simulink model "Simulation"  (R2020b)
settings: Solver=VariableStepAuto  StartTime=0.0  StopTime=15  RelTol=1e-3
values from neighbouring files (symbols this model uses):
  Ac = [0 1 0 0 ... (first row only)    [Model_Init.m]
  B1c = [0; 2*cf/m; 0; 2*lf*cf/iz]    [Model_Init.m]
  K = acker(Ac,B1c,kp)    [Model_Init.m]
  n_p = 30    [Model_Init.m]
  Ts = 0.1    [Model_Init.m]
  v0_ego = 13.9    [Model_Init.m]
undefined symbols (not defined in the file or in its folder): DiscIntNeverNeededParam
libraries: simulink x2
settings Model: Creator=Stage  LastModifiedBy=Stage

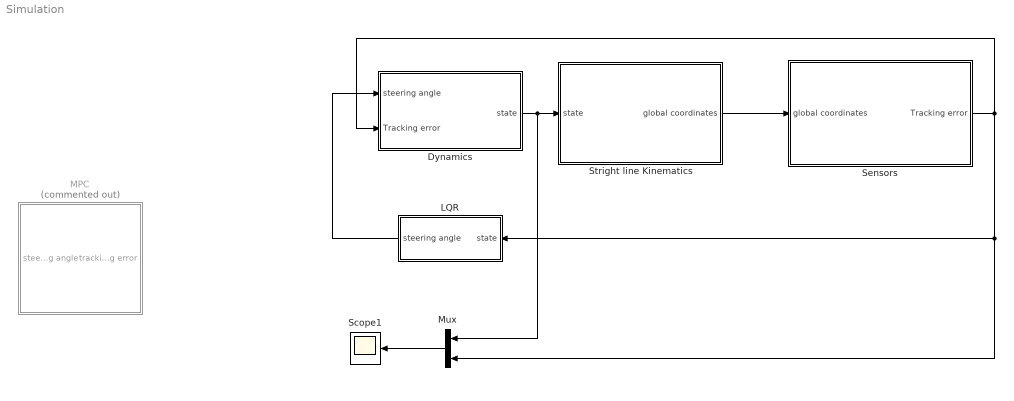
== system Simulation ==
  Dynamics : Subsystem
  "LQR " : Subsystem
  MPC : Subsystem  Commented=on
  Mux : Mux  Inputs=2
  Scope1 : Scope
  Sensors : Subsystem
  Stright line Kinematics : Subsystem
  wires:
  Stright line Kinematics/1(global coordinates) -> Sensors/1(global coordinates)
  Dynamics/1(state) -> Mux/1, Stright line Kinematics/1(state)
  Sensors/1(Tracking error) -> "LQR "/1(state), Mux/2, Dynamics/2(Tracking error)
  "LQR "/1(steering angle) -> Dynamics/1(steering angle)
  Mux/1 -> Scope1/1

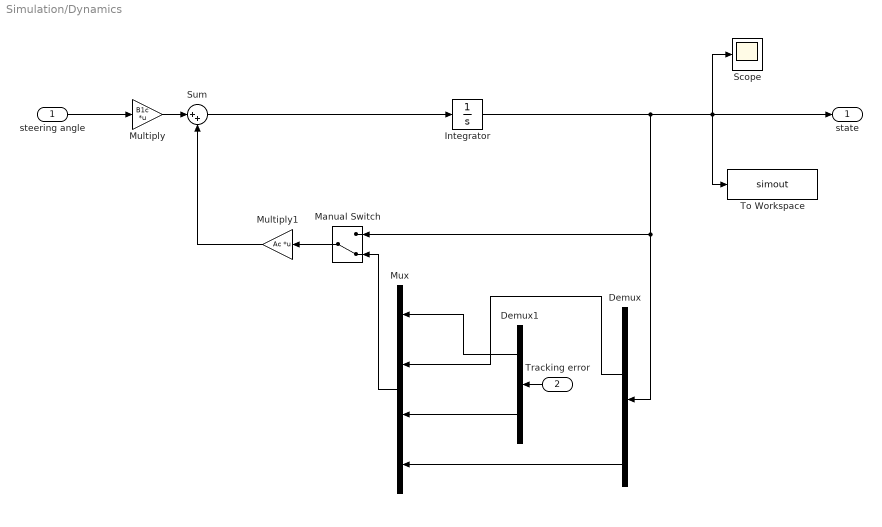
== system Simulation/Dynamics ==
  steering angle : Inport
  Tracking error : Inport  Port=2
  Demux : Demux
  Demux1 : Demux  Outputs=2
  Integrator : Integrator  InitialCondition=[1 0 0 0]
  Manual Switch : ManualSwitch  CurrentSetting=0
  Multiply : Gain  Gain=B1c  Multiplication=Matrix(K*u) (u vector)
  Multiply1 : Gain  Gain=Ac  Multiplication=Matrix(K*u) (u vector)
  Mux : Mux
  Scope : Scope
  Sum : Sum  Inputs=|++
  To Workspace : ToWorkspace  VariableName=simout  SampleTime=-1
  state : Outport
  wires:
  steering angle/1 -> Multiply/1
  Multiply/1 -> Sum/1
  Sum/1 -> Integrator/1
  Multiply1/1 -> Sum/2
  Manual Switch/1 -> Multiply1/1
  Mux/1 -> Manual Switch/2
  Tracking error/1 -> Demux1/1
  Integrator/1 -> Demux/1, Manual Switch/1, Scope/1, state/1, To Workspace/1
  Demux1/1 -> Mux/1
  Demux1/2 -> Mux/3
  Demux/2 -> Mux/2
  Demux/4 -> Mux/4

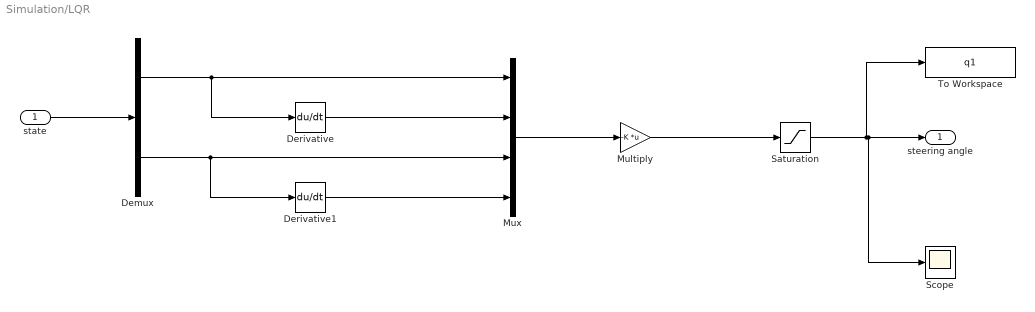
== system Simulation/LQR  ==
  state : Inport
  Demux : Demux  Outputs=2
  Derivative : Derivative
  Derivative1 : Derivative
  Multiply : Gain  Gain=-K  Multiplication=Matrix(K*u) (u vector)
  Mux : Mux
  Saturation : Saturate  UpperLimit=0.3  LowerLimit=-0.3
  Scope : Scope
  To Workspace : ToWorkspace  VariableName=q1  SaveFormat=Timeseries  SampleTime=-1
  steering angle : Outport
  wires:
  Multiply/1 -> Saturation/1
  Saturation/1 -> To Workspace/1, Scope/1, steering angle/1
  state/1 -> Demux/1
  Demux/1 -> Derivative/1, Mux/1
  Demux/2 -> Derivative1/1, Mux/3
  Derivative1/1 -> Mux/4
  Derivative/1 -> Mux/2
  Mux/1 -> Multiply/1

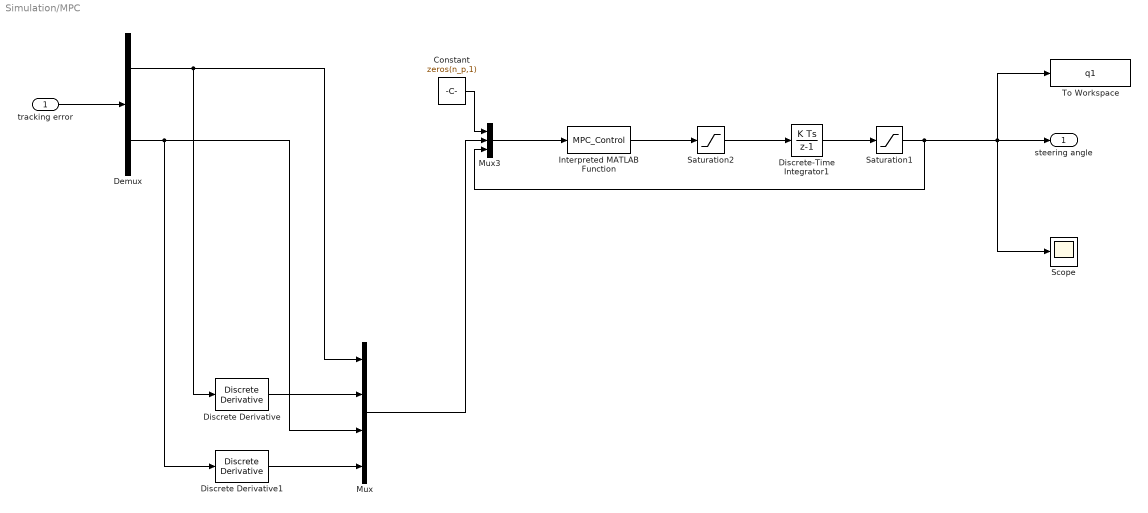
== system Simulation/MPC ==
  tracking error : Inport
  Constant : Constant  Value=zeros(n_p,1)
  Demux : Demux  Outputs=2
  Discrete Derivative : simulink/Discrete/Discrete Derivative  gainval=1.0  ICPrevScaledInput=10  OutMin=[]  OutMax=[]  OutDataType=fixdt(1, 16)  OutScaling=2^-10  DoSatur=off
  Discrete Derivative1 : simulink/Discrete/Discrete Derivative  gainval=1.0  ICPrevScaledInput=0.0  OutMin=[]  OutMax=[]  OutDataType=fixdt(1, 16)  OutScaling=2^-10  DoSatur=off
  Discrete-Time Integrator1 : DiscreteIntegrator  SampleTime=Ts  ICPrevOutput=DiscIntNeverNeededParam  ICPrevScaledInput=DiscIntNeverNeededParam
  Interpreted MATLAB Function : MATLABFcn  MATLABFcn=MPC_Control  OutputDimensions=1
  Mux : Mux
  Mux3 : Mux  Inputs=3
  Saturation1 : Saturate  UpperLimit=0.2  LowerLimit=-0.2
  Saturation2 : Saturate  UpperLimit=0.04  LowerLimit=-0.04
  Scope : Scope
  To Workspace : ToWorkspace  VariableName=q1  SampleTime=-1
  steering angle : Outport
  wires:
  Discrete-Time Integrator1/1 -> Saturation1/1
  Saturation1/1 -> Mux3/3, steering angle/1, Scope/1, To Workspace/1
  Mux3/1 -> Interpreted MATLAB Function/1
  Interpreted MATLAB Function/1 -> Saturation2/1
  Constant/1 -> Mux3/1
  tracking error/1 -> Demux/1
  Demux/1 -> Discrete Derivative/1, Mux/1
  Demux/2 -> Discrete Derivative1/1, Mux/3
  Mux/1 -> Mux3/2
  Discrete Derivative1/1 -> Mux/4
  Discrete Derivative/1 -> Mux/2
  Saturation2/1 -> Discrete-Time Integrator1/1

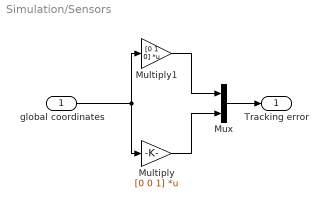
== system Simulation/Sensors ==
  global coordinates : Inport
  Multiply : Gain  Gain=[0 0 1]  Multiplication=Matrix(K*u) (u vector)
  Multiply1 : Gain  Gain=[0 1 0]  Multiplication=Matrix(K*u) (u vector)
  Mux : Mux  Inputs=2
  Tracking error : Outport
  wires:
  global coordinates/1 -> Multiply1/1, Multiply/1
  Multiply/1 -> Mux/2
  Multiply1/1 -> Mux/1
  Mux/1 -> Tracking error/1

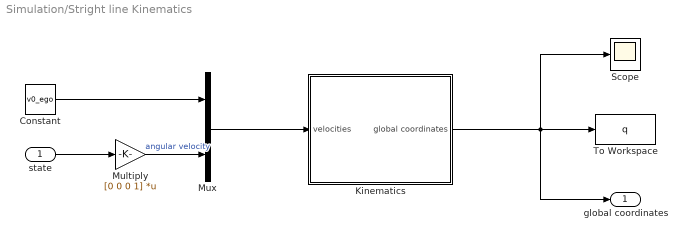
== system Simulation/Stright line Kinematics ==
  state : Inport
  Constant : Constant  Value=v0_ego
  "Kinematics " : Subsystem
  Multiply : Gain  Gain=[0 0 0 1]  Multiplication=Matrix(K*u) (u vector)
  Mux : Mux  Inputs=2
  Scope : Scope
  To Workspace : ToWorkspace  VariableName=q  SampleTime=-1
  global coordinates : Outport
  wires:
  Multiply/1 -> Mux/2  "angular velocity"
  Mux/1 -> "Kinematics "/1(velocities)
  "Kinematics "/1(global coordinates) -> To Workspace/1, global coordinates/1, Scope/1
  Constant/1 -> Mux/1
  state/1 -> Multiply/1

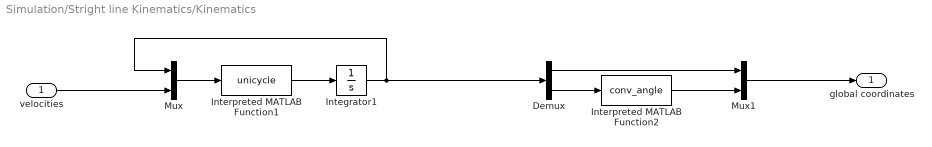
== system Simulation/Stright line Kinematics/Kinematics  ==
  velocities : Inport
  Demux : Demux  Outputs=[2 1]
  Integrator1 : Integrator  InitialCondition=[0; 1; 0]
  Interpreted MATLAB Function1 : MATLABFcn  MATLABFcn=unicycle
  Interpreted MATLAB Function2 : MATLABFcn  MATLABFcn=conv_angle
  Mux : Mux  Inputs=[3 2]
  Mux1 : Mux  Inputs=[2 1]
  global coordinates : Outport  VectorParamsAs1DForOutWhenUnconnected=off
  wires:
  Mux/1 -> Interpreted MATLAB Function1/1
  Interpreted MATLAB Function1/1 -> Integrator1/1
  Integrator1/1 -> Demux/1, Mux/1
  velocities/1 -> Mux/2
  Demux/2 -> Interpreted MATLAB Function2/1
  Interpreted MATLAB Function2/1 -> Mux1/2
  Demux/1 -> Mux1/1
  Mux1/1 -> global coordinates/1
